simulink model "quadExperiment"  (Simulink 9.0)
settings: Solver=ode45  StartTime=0.0  StopTime=50  MaxStep=0.01  RelTol=1e-3  EnableMultiTasking=on
libraries: simulink x1
settings Model: Creator=Alexey  LastModifiedBy=Stephen
settings DataIOCC: LimitDataPoints=on
settings OptimizationCC: ExpressionDepthLimit=2147483647
settings DebuggingCC: SolverPrmCheckMsg=warning  StateNameClashWarn=warning
settings GRTTargetCC: GeneratePreprocessorConditionals=Disable all
settings ConfigComp: CovSFcnEnable=off

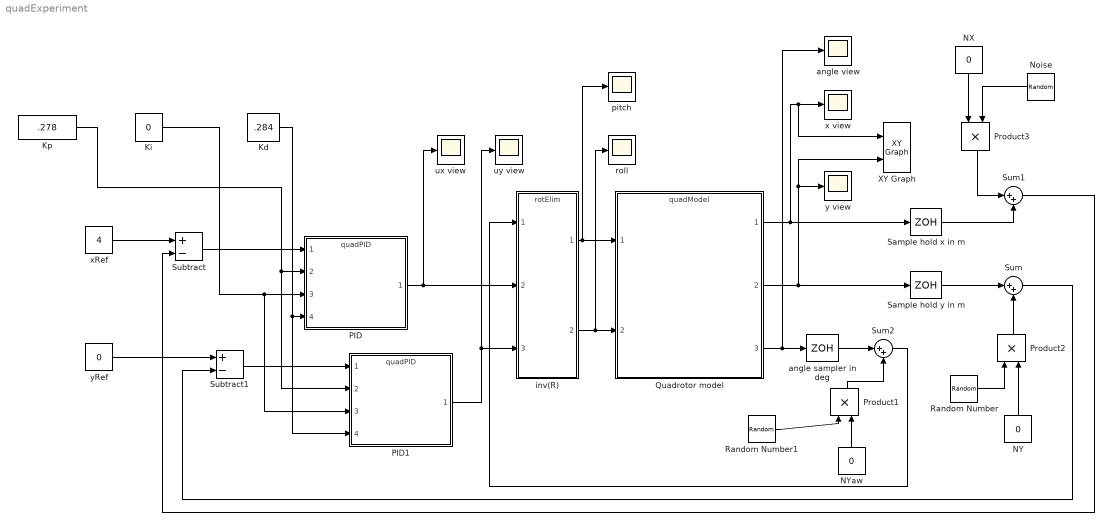
== system quadExperiment ==
  Kd : Constant  Value=.284
  Ki : Constant  Value=0
  Kp : Constant  Value=.278
  NX : Constant  Value=0
  NY : Constant  Value=0
  NYaw : Constant  Value=0
  Noise : RandomNumber  Variance=1e-4  SampleTime=0.1
  PID : ModelReference  ModelNameDialog=quadPID.mdl  SimulationMode=Normal  ModelReferenceVersion=1.28
  PID1 : ModelReference  ModelNameDialog=quadPID.mdl  SimulationMode=Normal  ModelReferenceVersion=1.28
  Product1 : Product  RndMeth=Zero
  Product2 : Product  RndMeth=Zero
  Product3 : Product  RndMeth=Zero
  Quadrotor model : ModelReference  ModelNameDialog=quadModel.mdl  SimulationMode=Normal  ModelReferenceVersion=1.38
  Random Number : RandomNumber  Variance=1e-4  Seed=2  SampleTime=0.1
  Random Number1 : RandomNumber  Seed=2  SampleTime=0.1
  Sample hold x in m : ZeroOrderHold  SampleTime=0.1
  Sample hold y in m : ZeroOrderHold  SampleTime=0.1
  Subtract : Sum  Inputs=+-
  Subtract1 : Sum  Inputs=+-
  Sum : Sum  Inputs=|++
  Sum1 : Sum  Inputs=|++
  Sum2 : Sum  Inputs=|++
  XY Graph : simulink/Sinks/XY Graph  xmin=-1  xmax=1  ymin=-1  ymax=1  st=-1
  angle sampler in deg : ZeroOrderHold  SampleTime=0.1
  angle view : Scope
  inv(R) : ModelReference  ModelNameDialog=rotElim.slx  SimulationMode=Normal  ModelReferenceVersion=1.10
  pitch : Scope
  roll : Scope
  ux view : Scope
  uy view : Scope
  x view : Scope
  xRef : Constant  Value=4
  y view : Scope
  yRef : Constant  Value=0
  wires:
  PID/1 -> inv(R)/2, ux view/1
  Subtract/1 -> PID/1
  xRef/1 -> Subtract/1
  yRef/1 -> Subtract1/1
  inv(R)/1 -> pitch/1, Quadrotor model/1
  Random Number/1 -> Product2/1
  NY/1 -> Product2/2
  Product2/1 -> Sum/2
  Quadrotor model/3 -> angle sampler in deg/1, angle view/1
  Quadrotor model/1 -> XY Graph/1, x view/1, Sample hold x in m/1
  Quadrotor model/2 -> Sample hold y in m/1, XY Graph/2, y view/1
  NX/1 -> Product3/1
  Sample hold x in m/1 -> Sum1/2
  Noise/1 -> Product3/2
  Product3/1 -> Sum1/1
  Sum/1 -> Subtract1/2
  Sample hold y in m/1 -> Sum/1
  Sum1/1 -> Subtract/2
  Random Number1/1 -> Product1/1
  NYaw/1 -> Product1/2
  angle sampler in deg/1 -> Sum2/1
  Product1/1 -> Sum2/2
  Sum2/1 -> inv(R)/1
  inv(R)/2 -> roll/1, Quadrotor model/2
  PID1/1 -> uy view/1, inv(R)/3
  Kp/1 -> PID1/2, PID/2
  Ki/1 -> PID/3, PID1/3
  Kd/1 -> PID1/4, PID/4
  Subtract1/1 -> PID1/1
